simulink model "WT_model"  (R2024a)
settings: Solver=FixedStepAuto  StartTime=0.0  StopTime=T_sim  FixedStep=dT  RelTol=1e-3
values from neighbouring files (symbols this model uses):
  b = 2e5    (= 200000)    [PMSG_test.m]    (also in PitchRegulated.m; StallRegulated.m; pitch_regulated.m; stall_regulated.m)
  Jeq = J_rotor+J_generator    (= 156004800)    [PMSG_test.m]    (also in PitchRegulated.m = 156000000; StallRegulated.m = 156000000; pitch_regulated.m = 156000000; stall_regulated.m = 156000000)
  lambda_opt = lambda_sweep(find(~(Cp_map(:,1) - max(Cp_map(:,1)))))    [PMSG_test.m]    (also in PitchRegulated.m; pitch_regulated.m)
  omega_rotor_0 = Vw_ramp(1)*lambda_opt/R_rotor    [PMSG_test.m]    (also in PitchRegulated.m; StallRegulated.m = 0.1; pitch_regulated.m; stall_regulated.m = 0.1)
  R_rotor = 178.3/2    (= 89.15)    [PMSG_test.m]    (also in PitchRegulated.m; StallRegulated.m; pitch_regulated.m; stall_regulated.m)
  rho_air = 1.225    [PMSG_test.m]    (also in PitchRegulated.m; StallRegulated.m; pitch_regulated.m; stall_regulated.m)
  Trated = Cp_opt/lambda_opt*0.5*rho_air*A_rotor.*V_rated^2*R_rotor    [PMSG_test.m]    (also in PitchRegulated.m; pitch_regulated.m)
  V_ci = 4    [PMSG_test.m]    (also in PitchRegulated.m; StallRegulated.m; pitch_regulated.m; stall_regulated.m)
  V_co = 25    [PMSG_test.m]    (also in PitchRegulated.m; StallRegulated.m; pitch_regulated.m; stall_regulated.m)
  V_rated = 11.4    [PMSG_test.m]    (also in PitchRegulated.m; StallRegulated.m; pitch_regulated.m; stall_regulated.m)
  Vw_timeseries = timeseries(Vw_ramp',time')    [PMSG_test.m]    (also in PitchRegulated.m; StallRegulated.m; pitch_regulated.m; stall_regulated.m)
libraries: slpidlib x3
settings Model: Creator=marti  LastModifiedBy=Andrea
settings DebuggingCC: AlgebraicLoopMsg=none
settings RTWCC: GPUComputeCapability=3.5

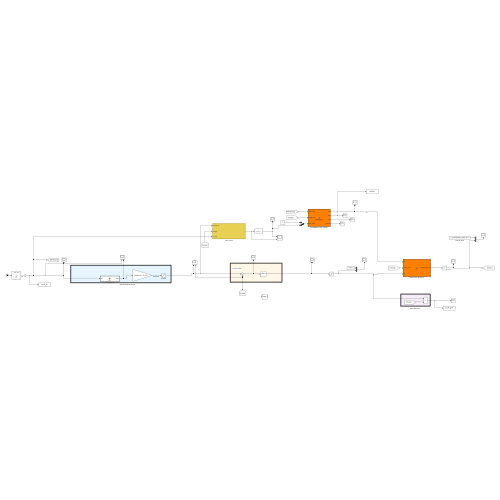
[thumbnail: Simulink's stored preview of the top-level diagram]
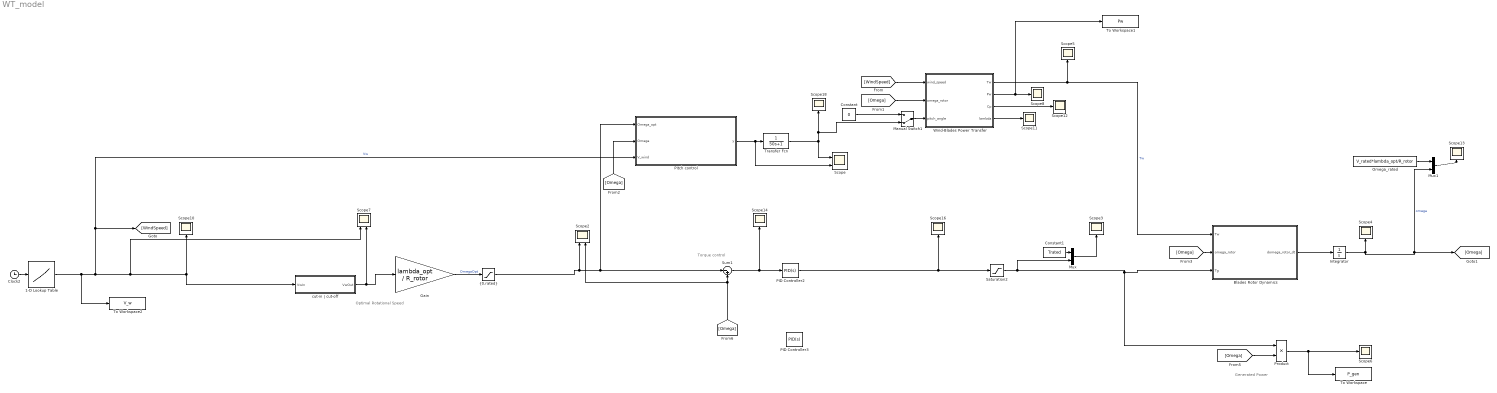
== system WT_model ==
  note: Torque control
  note: Generated Power
  note: Optimal Rotational Speed
  1-D Lookup Table : Lookup_n-D  NumberOfTableDimensions=1  BreakpointsForDimension1=Vw_timeseries.Time  Table=Vw_timeseries.Data  InternalRulePriority=Speed  RndMeth=Simplest
  Blades Rotor Dynamics : MATLAB Function  TreatAsAtomicUnit=on
  Clock2 : Clock
  Constant : Constant  Value=0
  Constant1 : Constant  Value=Trated
  Gain : Gain  Gain=lambda_opt / R_rotor
  Integrator : Integrator  InitialCondition=omega_rotor_0
  Manual Switch1 : ManualSwitch  CurrentSetting=0
  Mux : Mux  Inputs=2
  Mux1 : Mux  Inputs=2
  Omega_rated : Constant  Value=V_rated*lambda_opt/R_rotor
  PID Controller2 : slpidlib/PID Controller  Controller=PID  Form=Parallel  TimeDomain=Continuous-time  UseExternalTs=off  SampleTime=-1  IntegratorMethod=Forward Euler  FilterMethod=Forward Euler  ControllerParametersSource=internal  P=92825719.0349632  I=13263093.1982927  UseKiTs=off  D=32692738.6851362  UseExternalDerivativeSource=off  N=0.939630797387095  UseFilter=on  TunerSelectOption=Transfer Function Based (PID Tuner App)  InitialConditionSource=internal  InitialConditionForIntegrator=0  InitialConditionForFilter=0  DifferentiatorICPrevScaledInput=0  ExternalReset=none  TrackingMode=off  Kt=1  LimitOutput=off  SatLimitsSource=internal  UpperSaturationLimit=inf  LowerSaturationLimit=-inf  LinearizeAsGain=on  AntiWindupMode=none  Kb=1  LimitIntegrator=off  UpperIntegratorSaturationLimit=inf  LowerIntegratorSaturationLimit=-inf  POutMin=[]  POutMax=[]  IOutMin=[]  IOutMax=[]  DOutMin=[]  DOutMax=[]  NOutMin=[]  NOutMax=[]  SumOutMin=[]  SumOutMax=[]  SaturationOutMin=[]  SaturationOutMax=[]  PParamMin=[]  PParamMax=[]  IParamMin=[]  IParamMax=[]  DParamMin=[]  DParamMax=[]  NParamMin=[]  NParamMax=[]  KbParamMin=[]  KbParamMax=[]  KtParamMin=[]  KtParamMax=[]  KbOutMin=[]  KbOutMax=[]  KtOutMin=[]  KtOutMax=[]  IntegratorOutMin=[]  IntegratorOutMax=[]  FilterOutMin=[]  FilterOutMax=[]  SumI1OutMin=[]  SumI1OutMax=[]  SumI2OutMin=[]  SumI2OutMax=[]  SumI3OutMin=[]  SumI3OutMax=[]  SumI4OutMin=[]  SumI4OutMax=[]  SumDOutMin=[]  SumDOutMax=[]  DifferentiatorOutMin=[]  DifferentiatorOutMax=[]  FilterDiffOutCoefMin=[]  FilterDiffOutCoefMax=[]  ReciprocalOutMin=[]  ReciprocalOutMax=[]  SumDenOutMin=[]  SumDenOutMax=[]  SumNumOutMin=[]  SumNumOutMax=[]  DivideOutMin=[]  DivideOutMax=[]  UdiffTsProdOutMin=[]  UdiffTsProdOutMax=[]  NTsProdOutMin=[]  NTsProdOutMax=[]  UintegralTsProdOutMin=[]  UintegralTsProdOutMax=[]  UngainTsProdOutMin=[]  UngainTsProdOutMax=[]  ClampingZeroOutDataTypeStr=Inherit: Inherit via back propagation  ClampingZeroOutMin=[]  ClampingZeroOutMax=[]  FilterDenConstantOutDataTypeStr=Inherit: Inherit via back propagation  FilterDenConstantOutMin=[]  FilterDenConstantOutMax=[]  PCopyOutDataTypeStr=Inherit: Inherit via back propagation  PCopyOutMin=[]  PCopyOutMax=[]  NCopyOutDataTypeStr=Inherit: Inherit via back propagation  NCopyOutMin=[]  NCopyOutMax=[]  IntegratorContinuousStateAttributes=''  IntegratorStateMustResolveToSignalObject=off  IntegratorRTWStateStorageClass=Auto  FilterContinuousStateAttributes=''  FilterStateMustResolveToSignalObject=off  FilterRTWStateStorageClass=Auto  ParallelPVariant=InternalParameters  IdealPVariant=Disabled  IVariant=InternalParameters  DVariant=InternalParameters  IntegratorVariant=Continuous  SatVariant=Disabled  AWVariant=Passthrough  PCopyVariant=Disabled  TRVariant=Disabled  FdbkBlocksVariant=Forward  IdealPFdbkVariant=Disabled  SatFdbkVariant=Disabled  DerivativeFilterVariant=ContFilter  NVariant=InternalParameters  NCopyVariant=Disabled  FilterICVariant=InternalICsFilter  IntegratorICVariant=InternalICs  ExternalResetVariant=Disabled  TRSumVariant=Passthrough  SumFdbkVariant=Disabled  SumVariant=Sum_PID  TsampFilterVariant=InternalTs  TsampNgainVariant=Passthrough  TsampIntegralVariant=Disabled_SignalSpec  ExternalSaturationOutDataTypeStr=Inherit: Same as second input  DerivativeSourceVariant=ErrorSignal
  PID Controller3 : slpidlib/PID Controller  Controller=PID  Form=Parallel  TimeDomain=Continuous-time  UseExternalTs=off  SampleTime=-1  IntegratorMethod=Forward Euler  FilterMethod=Forward Euler  ControllerParametersSource=internal  P=52503810.0885907  I=14518412.7007273  UseKiTs=off  D=5217462.76167334  UseExternalDerivativeSource=off  N=5.66897900590121  UseFilter=on  TunerSelectOption=Transfer Function Based (PID Tuner App)  InitialConditionSource=internal  InitialConditionForIntegrator=0  InitialConditionForFilter=0  DifferentiatorICPrevScaledInput=0  ExternalReset=none  TrackingMode=off  Kt=1  LimitOutput=off  SatLimitsSource=internal  UpperSaturationLimit=inf  LowerSaturationLimit=-inf  LinearizeAsGain=on  AntiWindupMode=none  Kb=1  LimitIntegrator=off  UpperIntegratorSaturationLimit=inf  LowerIntegratorSaturationLimit=-inf  POutMin=[]  POutMax=[]  IOutMin=[]  IOutMax=[]  DOutMin=[]  DOutMax=[]  NOutMin=[]  NOutMax=[]  SumOutMin=[]  SumOutMax=[]  SaturationOutMin=[]  SaturationOutMax=[]  PParamMin=[]  PParamMax=[]  IParamMin=[]  IParamMax=[]  DParamMin=[]  DParamMax=[]  NParamMin=[]  NParamMax=[]  KbParamMin=[]  KbParamMax=[]  KtParamMin=[]  KtParamMax=[]  KbOutMin=[]  KbOutMax=[]  KtOutMin=[]  KtOutMax=[]  IntegratorOutMin=[]  IntegratorOutMax=[]  FilterOutMin=[]  FilterOutMax=[]  SumI1OutMin=[]  SumI1OutMax=[]  SumI2OutMin=[]  SumI2OutMax=[]  SumI3OutMin=[]  SumI3OutMax=[]  SumI4OutMin=[]  SumI4OutMax=[]  SumDOutMin=[]  SumDOutMax=[]  DifferentiatorOutMin=[]  DifferentiatorOutMax=[]  FilterDiffOutCoefMin=[]  FilterDiffOutCoefMax=[]  ReciprocalOutMin=[]  ReciprocalOutMax=[]  SumDenOutMin=[]  SumDenOutMax=[]  SumNumOutMin=[]  SumNumOutMax=[]  DivideOutMin=[]  DivideOutMax=[]  UdiffTsProdOutMin=[]  UdiffTsProdOutMax=[]  NTsProdOutMin=[]  NTsProdOutMax=[]  UintegralTsProdOutMin=[]  UintegralTsProdOutMax=[]  UngainTsProdOutMin=[]  UngainTsProdOutMax=[]  ClampingZeroOutDataTypeStr=Inherit: Inherit via back propagation  ClampingZeroOutMin=[]  ClampingZeroOutMax=[]  FilterDenConstantOutDataTypeStr=Inherit: Inherit via back propagation  FilterDenConstantOutMin=[]  FilterDenConstantOutMax=[]  PCopyOutDataTypeStr=Inherit: Inherit via back propagation  PCopyOutMin=[]  PCopyOutMax=[]  NCopyOutDataTypeStr=Inherit: Inherit via back propagation  NCopyOutMin=[]  NCopyOutMax=[]  IntegratorContinuousStateAttributes=''  IntegratorStateMustResolveToSignalObject=off  IntegratorRTWStateStorageClass=Auto  FilterContinuousStateAttributes=''  FilterStateMustResolveToSignalObject=off  FilterRTWStateStorageClass=Auto  ParallelPVariant=InternalParameters  IdealPVariant=Disabled  IVariant=InternalParameters  DVariant=InternalParameters  IntegratorVariant=Continuous  SatVariant=Disabled  AWVariant=Passthrough  PCopyVariant=Disabled  TRVariant=Disabled  FdbkBlocksVariant=Forward  IdealPFdbkVariant=Disabled  SatFdbkVariant=Disabled  DerivativeFilterVariant=ContFilter  NVariant=InternalParameters  NCopyVariant=Disabled  FilterICVariant=InternalICsFilter  IntegratorICVariant=InternalICs  ExternalResetVariant=Disabled  TRSumVariant=Passthrough  SumFdbkVariant=Disabled  SumVariant=Sum_PID  TsampFilterVariant=InternalTs  TsampNgainVariant=Passthrough  TsampIntegralVariant=Disabled_SignalSpec  ExternalSaturationOutDataTypeStr=Inherit: Same as second input  DerivativeSourceVariant=ErrorSignal
  Pitch control : Subsystem
  Product : Product
  Saturation2 : Saturate  UpperLimit=Trated  LowerLimit=-Inf
  Scope : Scope  NumInputPorts=2
  Scope{3..6,8,10..14,16,18} (12 alike) : Scope
  Scope2 : Scope  NumInputPorts=2
  Scope7 : Scope  NumInputPorts=2
  Sum1 : Sum  Inputs=|-+
  To Workspace : ToWorkspace  VariableName=P_gen  SampleTime=-1
      settings: Save2DSignal=2-D array (concatenate along first dimension)
  To Workspace1 : ToWorkspace  VariableName=Pw  SampleTime=-1
      settings: Save2DSignal=2-D array (concatenate along first dimension)
  To Workspace2 : ToWorkspace  VariableName=V_w  SampleTime=-1
      settings: Save2DSignal=2-D array (concatenate along first dimension)
  Transfer Fcn : TransferFcn  Denominator=[50 1]
  Wind-Blades Power Transfer : MATLAB Function  TreatAsAtomicUnit=on
  cut-in | cut-off : MATLAB Function  TreatAsAtomicUnit=on
  "{0,rated}" : Saturate  UpperLimit=V_rated*lambda_opt/R_rotor  LowerLimit=0
  wires:
  Gain/1 -> "{0,rated}"/1  "OmegaOpt"
  [WindSpeed] -> Wind-Blades Power Transfer/1(wind_speed)
  Wind-Blades Power Transfer/1(Tw) -> Blades Rotor Dynamics/1(Tw), Scope5/1  "Tw"
  Blades Rotor Dynamics/1(domega_rotor_dt) -> Integrator/1
  Integrator/1 -> [Omega], Mux1/2, Scope4/1  "omega"
  [Omega] -> Wind-Blades Power Transfer/2(omega_rotor)
  [Omega] -> Blades Rotor Dynamics/2(omega_rotor)
  [Omega] -> Product/2
  Product/1 -> To Workspace/1, Scope6/1
  1-D Lookup Table/1 -> Scope7/1, cut-in | cut-off/1(VwIn), Scope10/1, Pitch control/3(V_wind), [WindSpeed], To Workspace2/1  "Vw"
  "{0,rated}"/1 -> Scope2/1, Pitch control/1(Omega_opt), Sum1/1
  Wind-Blades Power Transfer/4(lambda) -> Scope11/1
  Wind-Blades Power Transfer/3(Cp) -> Scope12/1
  Manual Switch1/1 -> Wind-Blades Power Transfer/3(pitch_angle)
  Constant/1 -> Manual Switch1/1
  [Omega] -> Scope2/2, Sum1/2
  Wind-Blades Power Transfer/2(Pw) -> To Workspace1/1, Scope8/1
  Clock2/1 -> 1-D Lookup Table/1
  Constant1/1 -> Mux/1
  Mux/1 -> Scope3/1
  Omega_rated/1 -> Mux1/1
  Mux1/1 -> Scope13/1
  Sum1/1 -> PID Controller2/1, Scope14/1
  Saturation2/1 -> Blades Rotor Dynamics/3(Tg), Product/1, Mux/2
  [Omega] -> Pitch control/2(Omega)
  PID Controller2/1 -> Scope16/1, Saturation2/1
  cut-in | cut-off/1(VwOut) -> Scope7/2, Gain/1
  Pitch control/1(y) -> Scope/2, Transfer Fcn/1
  Transfer Fcn/1 -> Scope/1, Scope18/1, Manual Switch1/2

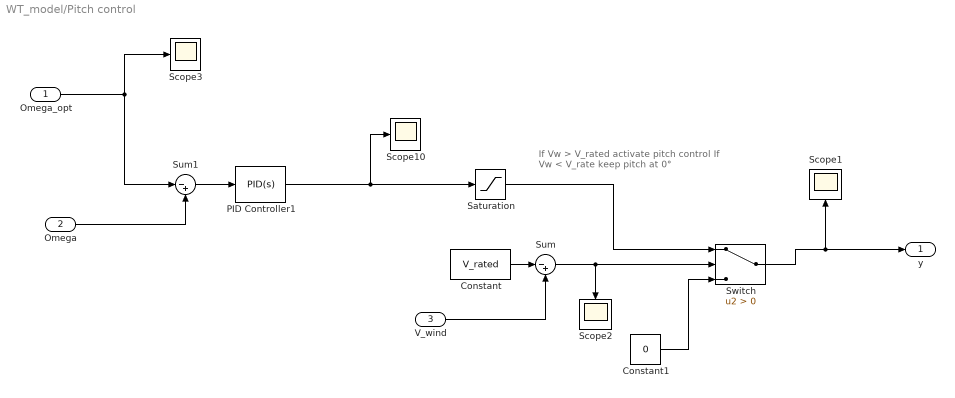
== system WT_model/Pitch control ==
  note: If Vw  >  V_rated activate pitch control
      | If Vw < V_rate keep pitch at 0°
  Omega_opt : Inport
  Omega : Inport  Port=2
  V_wind : Inport  Port=3
  Constant : Constant  Value=V_rated
  Constant1 : Constant  Value=0
  PID Controller1 : slpidlib/PID Controller  Controller=PID  Form=Parallel  TimeDomain=Continuous-time  UseExternalTs=off  SampleTime=-1  IntegratorMethod=Forward Euler  FilterMethod=Forward Euler  ControllerParametersSource=internal  P=1700  I=5  UseKiTs=off  D=0  UseExternalDerivativeSource=off  N=100  UseFilter=on  TunerSelectOption=Transfer Function Based (PID Tuner App)  InitialConditionSource=internal  InitialConditionForIntegrator=0  InitialConditionForFilter=0  DifferentiatorICPrevScaledInput=0  ExternalReset=none  TrackingMode=off  Kt=1  LimitOutput=off  SatLimitsSource=internal  UpperSaturationLimit=inf  LowerSaturationLimit=-inf  LinearizeAsGain=on  AntiWindupMode=none  Kb=1  LimitIntegrator=off  UpperIntegratorSaturationLimit=inf  LowerIntegratorSaturationLimit=-inf  POutMin=[]  POutMax=[]  IOutMin=[]  IOutMax=[]  DOutMin=[]  DOutMax=[]  NOutMin=[]  NOutMax=[]  SumOutMin=[]  SumOutMax=[]  SaturationOutMin=[]  SaturationOutMax=[]  PParamMin=[]  PParamMax=[]  IParamMin=[]  IParamMax=[]  DParamMin=[]  DParamMax=[]  NParamMin=[]  NParamMax=[]  KbParamMin=[]  KbParamMax=[]  KtParamMin=[]  KtParamMax=[]  KbOutMin=[]  KbOutMax=[]  KtOutMin=[]  KtOutMax=[]  IntegratorOutMin=[]  IntegratorOutMax=[]  FilterOutMin=[]  FilterOutMax=[]  SumI1OutMin=[]  SumI1OutMax=[]  SumI2OutMin=[]  SumI2OutMax=[]  SumI3OutMin=[]  SumI3OutMax=[]  SumI4OutMin=[]  SumI4OutMax=[]  SumDOutMin=[]  SumDOutMax=[]  DifferentiatorOutMin=[]  DifferentiatorOutMax=[]  FilterDiffOutCoefMin=[]  FilterDiffOutCoefMax=[]  ReciprocalOutMin=[]  ReciprocalOutMax=[]  SumDenOutMin=[]  SumDenOutMax=[]  SumNumOutMin=[]  SumNumOutMax=[]  DivideOutMin=[]  DivideOutMax=[]  UdiffTsProdOutMin=[]  UdiffTsProdOutMax=[]  NTsProdOutMin=[]  NTsProdOutMax=[]  UintegralTsProdOutMin=[]  UintegralTsProdOutMax=[]  UngainTsProdOutMin=[]  UngainTsProdOutMax=[]  ClampingZeroOutDataTypeStr=Inherit: Inherit via back propagation  ClampingZeroOutMin=[]  ClampingZeroOutMax=[]  FilterDenConstantOutDataTypeStr=Inherit: Inherit via back propagation  FilterDenConstantOutMin=[]  FilterDenConstantOutMax=[]  PCopyOutDataTypeStr=Inherit: Inherit via back propagation  PCopyOutMin=[]  PCopyOutMax=[]  NCopyOutDataTypeStr=Inherit: Inherit via back propagation  NCopyOutMin=[]  NCopyOutMax=[]  IntegratorContinuousStateAttributes=''  IntegratorStateMustResolveToSignalObject=off  IntegratorRTWStateStorageClass=Auto  FilterContinuousStateAttributes=''  FilterStateMustResolveToSignalObject=off  FilterRTWStateStorageClass=Auto  ParallelPVariant=InternalParameters  IdealPVariant=Disabled  IVariant=InternalParameters  DVariant=InternalParameters  IntegratorVariant=Continuous  SatVariant=Disabled  AWVariant=Passthrough  PCopyVariant=Disabled  TRVariant=Disabled  FdbkBlocksVariant=Forward  IdealPFdbkVariant=Disabled  SatFdbkVariant=Disabled  DerivativeFilterVariant=ContFilter  NVariant=InternalParameters  NCopyVariant=Disabled  FilterICVariant=InternalICsFilter  IntegratorICVariant=InternalICs  ExternalResetVariant=Disabled  TRSumVariant=Passthrough  SumFdbkVariant=Disabled  SumVariant=Sum_PID  TsampFilterVariant=InternalTs  TsampNgainVariant=Passthrough  TsampIntegralVariant=Disabled_SignalSpec  ExternalSaturationOutDataTypeStr=Inherit: Same as second input  DerivativeSourceVariant=ErrorSignal
  Saturation : Saturate  UpperLimit=30  LowerLimit=0
  Scope{1..3,10} (4 alike) : Scope
  Sum : Sum  Inputs=|-+
  Sum1 : Sum  Inputs=|-+
  Switch : Switch  Criteria=u2 > Threshold  SaturateOnIntegerOverflow=off  InputSameDT=off
  y : Outport
  wires:
  PID Controller1/1 -> Saturation/1, Scope10/1
  Omega/1 -> Sum1/2
  Omega_opt/1 -> Sum1/1, Scope3/1
  Sum1/1 -> PID Controller1/1
  Saturation/1 -> Switch/1
  Constant1/1 -> Switch/3
  Sum/1 -> Switch/2, Scope2/1
  V_wind/1 -> Sum/2
  Constant/1 -> Sum/1
  Switch/1 -> y/1, Scope1/1

== matlab function WT_model/cut-in | cut-off ==
  data: VwIn input; VwOut output; V_ci parameter; V_co parameter; V_rated parameter
function VwOut = fcn(VwIn,V_ci, V_co,V_rated)
if VwIn < V_ci
    VwOut = 0;
elseif VwIn >= V_ci && VwIn < V_co
    VwOut = VwIn;
else 
    VwOut = 0;
end

== matlab function WT_model/Blades Rotor Dynamics ==
  data: Tw input; omega_rotor input; domega_rotor_dt output; Tg input; Jeq parameter; b parameter
  function domega_rotor_dt = fcn(Tw,omega_rotor,Tg,Jeq,b)

% Blades rotor shaft torques equilibrium:
% domega/dt * Jeq + b * omega = T_wind - T_generator

domega_rotor_dt = (Tw-Tg-b*omega_rotor)/Jeq;

== matlab function WT_model/Wind-Blades Power Transfer ==
  data: wind_speed input; Tw output; omega_rotor input; pitch_angle input; R_rotor parameter; rho_air parameter; Pw output; Cp output; lambda output
function [Tw,Pw,Cp,lambda]   = WindTorque(wind_speed,omega_rotor,pitch_angle,R_rotor,rho_air)

fake_zero = 1e-6;
% Power Factor
lambda = omega_rotor*R_rotor/wind_speed;
Cp = PowerFactor(lambda,pitch_angle);
if Cp < fake_zero
    Cp = fake_zero;
end

% Wind power
Pw = 0.5 * rho_air * (pi * R_rotor^2) * Cp * wind_speed^3;

% Wind torque
Tw = Pw / omega_rotor;
